simulink model "lqr_tracking_backup"  (R2017a)
settings: Solver=ode5  StartTime=0.0  StopTime=50  FixedStep=Ts  RelTol=1e-3  EnableMultiTasking=on
values from neighbouring files (symbols this model uses):
  Ki_lqr = [0 0 0.1 0 0 -0.1 0 0 8.66025403784 0 0 0 ... (16 elements, 4x4)]    [K_lqr.mat]
  Kx_lqr = [0 0 0.263619393691 0 0 -0.257300038922 0 0 13.6588017709 0 0 0 ... (48 elements, 4x12)]    [K_lqr.mat]
undefined symbols (not defined in the file or in its folder): B_ENU_inv, gra, KT, mass, sigbuilder_block
settings Model: Creator=dtnguyen  LastModifiedBy=ducnguyen
settings DataIOCC: LimitDataPoints=on  SaveFormat=Array
settings OptimizationCC: DefaultParameterBehavior=Inlined  UseFloatMulNetSlope=on  InlineInvariantSignals=on  PassReuseOutputArgsThreshold=0  EfficientFloat2IntCast=on
settings DebuggingCC: ParameterTunabilityLossMsg=error  SFUnexpectedBacktrackingDiag=warning  SFNoUnconditionalDefaultTransitionDiag=warning  SFExecutionAtInitializationDiag=none
settings HardwareCC: ProdBitPerPointer=32  ProdBitPerSizeT=32  ProdBitPerPtrDiffT=32  ProdLargestAtomicFloat=None  ProdIntDivRoundTo=Undefined  ProdEndianess=Unspecified  ProdWordSize=32  ProdHWDeviceType=32-bit Generic
settings ModelReferenceCC: PropagateSignalLabelsOutOfModel=off
settings RTWCC: PackageGeneratedCodeAndArtifacts=on  PackageName=myCodeExport  GenerateReport=on  Toolchain=Catkin  BuildConfiguration=Faster Runs  LaunchReport=on  TargetLang=C++  CheckMdlBeforeBuild=Warning
settings CodeAppCC: ForceParamTrailComments=on  OperatorAnnotations=on  MATLABSourceComments=on
settings GRTTargetCC: TargetLangStandard=C++03 (ISO)  MatFileLogging=off  MultiInstanceERTCode=on  CodeInterfacePackaging=C++ class
settings ConfigComp: CovMetricSettings=dw  CovHtmlReporting=on  CovSaveCumulativeToWorkspaceVar=on  CovSaveSingleToWorkspaceVar=on  CovExternalEMLEnable=off

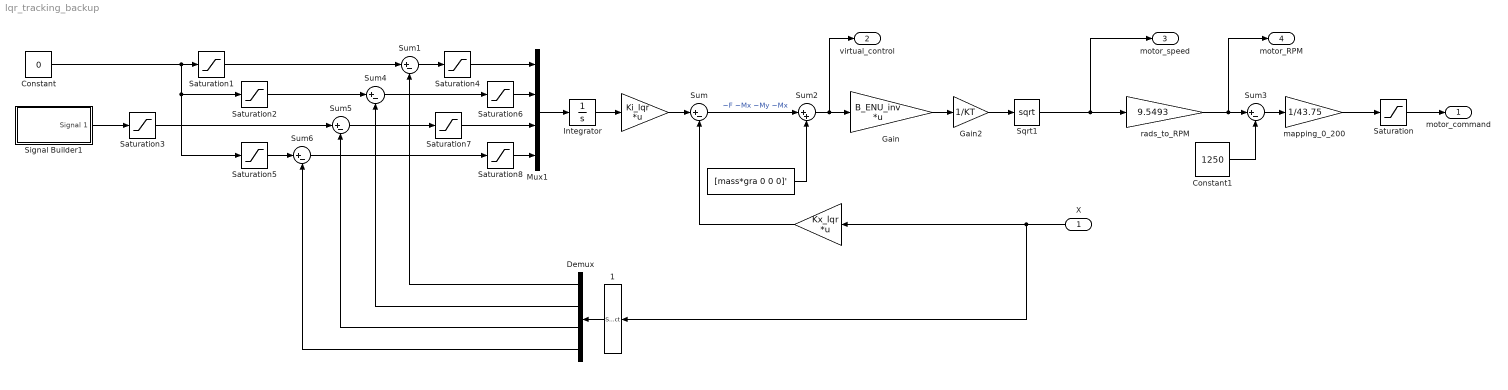
== system lqr_tracking_backup ==
  X : Inport  PortDimensions=12
  " " : Gain  Gain=Ki_lqr  Multiplication=Matrix(K*u)
  "              " : Constant  Value=[mass*gra 0 0 0]'
  "                   " : Gain  Gain=Kx_lqr  Multiplication=Matrix(K*u)
  "                    1" : Selector  InputPortWidth=12  IndexOptions=Index vector (dialog)  Indices=[1 2 3 9]  OutputSizes=1
  Constant : Constant  Value=0
  Constant1 : Constant  Value=1250  VectorParams1D=off  SampleTime=-1
  Demux : Demux
  Gain : Gain  Gain=B_ENU_inv  Multiplication=Matrix(K*u)
  Gain2 : Gain  Gain=1/KT
  Integrator : Integrator  InitialCondition=[0 0 0 0]'
  Mux1 : Mux
  Saturation : Saturate  UpperLimit=200  LowerLimit=0
  Saturation1 : Saturate  UpperLimit=2  LowerLimit=-2
  Saturation2 : Saturate  UpperLimit=2  LowerLimit=-2
  Saturation3 : Saturate  UpperLimit=1.75  LowerLimit=0
  Saturation4 : Saturate  UpperLimit=1  LowerLimit=-1
  Saturation5 : Saturate  UpperLimit=2*pi  LowerLimit=-2*pi
  Saturation6 : Saturate  UpperLimit=1  LowerLimit=-1
  Saturation7 : Saturate
  Saturation8 : Saturate  UpperLimit=pi/4  LowerLimit=-pi/4
  Signal Builder1 : Subsystem  Tag=STV Subsys  LoadFcn=sigbuilder_block('load');  StartFcn=sigbuilder_block('start');  StopFcn=sigbuilder_block('stop');  ClipboardFcn=sigbuilder_block('clipboard');  mask(Sigbuilder block){tuvar=[0:10]}
      mask help: Simulink:masks:SigbuilderBlock_MD
      mask init:
      | if ~strcmp(get_param(bdroot(gcbh),'SimulationStatus'),'stopped') tuvar = sigbuilder_block('maskInit'); end
      settings: CopyFcn=sigbuilder_block('copy');  DeleteFcn=sigbuilder_block('delete');  ModelCloseFcn=sigbuilder_block('modelClose');  PreSaveFcn=sigbuilder_block('preSave');  PauseFcn=sigbuilder_block('pause');  ContinueFcn=sigbuilder_block('continue');  NameChangeFcn=sigbuilder_block('namechange');  OpenFcn=sigbuilder_block('open',[425.25 198.75 556.5 403.5 ]);  CloseFcn=sigbuilder_block('close');
      mask Display: plot(0, 0, 100, 100,[2, 2, 32, 32, 2], [68, 8, 8, 68, 68],[32, 2], [38, 38], [32, 19, 2],[53, 60, 44], [32, 17, 17, 2],[16, 16, 31, 31]);txt = getActiveGroup(gcbh);text(2, 100, txt,'verticalAlignment', 'top');
  Sqrt1 : Sqrt  SaturateOnIntegerOverflow=on
  Sum{,1,3..6} (6 alike) : Sum  Inputs=|+-
  Sum2 : Sum  Inputs=|++
  mapping_0_200 : Gain  Gain=1/43.75
  rads_to_RPM : Gain  Gain=9.5493
  motor_command : Outport  PortDimensions=6
  virtual_control : Outport  Port=2  PortDimensions=4
  motor_speed : Outport  Port=3  PortDimensions=6
  motor_RPM : Outport  Port=4  PortDimensions=6
  wires:
  Gain2/1 -> Sqrt1/1
  X/1 -> "                   "/1, "                    1"/1
  Mux1/1 -> Integrator/1
  " "/1 -> Sum/1
  Integrator/1 -> " "/1
  "                   "/1 -> Sum/2
  Gain/1 -> Gain2/1
  Sum2/1 -> Gain/1, virtual_control/1
  Sum/1 -> Sum2/1  "~F ~Mx ~My ~Mx"
  "              "/1 -> Sum2/2
  Constant1/1 -> Sum3/2
  rads_to_RPM/1 -> Sum3/1, motor_RPM/1
  Sum3/1 -> mapping_0_200/1
  mapping_0_200/1 -> Saturation/1
  Saturation/1 -> motor_command/1
  Saturation1/1 -> Sum1/1
  Sum1/1 -> Saturation4/1
  Sum4/1 -> Saturation6/1
  Sum5/1 -> Saturation7/1
  Sum6/1 -> Saturation8/1
  "                    1"/1 -> Demux/1
  Demux/1 -> Sum1/2
  Demux/2 -> Sum4/2
  Demux/3 -> Sum5/2
  Demux/4 -> Sum6/2
  Saturation2/1 -> Sum4/1
  Saturation3/1 -> Sum5/1
  Constant/1 -> Saturation1/1, Saturation5/1, Saturation2/1
  Saturation4/1 -> Mux1/1
  Saturation5/1 -> Sum6/1
  Saturation6/1 -> Mux1/2
  Saturation7/1 -> Mux1/3
  Saturation8/1 -> Mux1/4
  Sqrt1/1 -> rads_to_RPM/1, motor_speed/1
  Signal Builder1/1(Signal 1) -> Saturation3/1

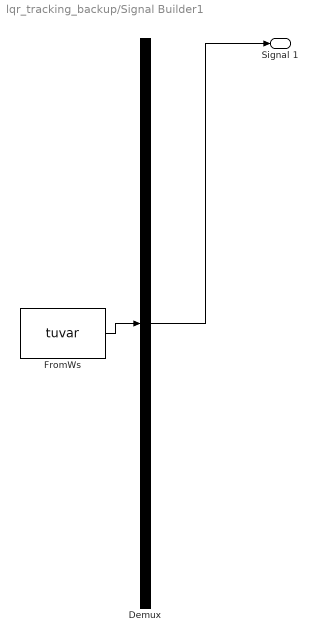
== system lqr_tracking_backup/Signal Builder1 ==
  Demux : Demux  Tag=STV Demux  Outputs=1
  FromWs : FromWorkspace  Tag=STV FromWs  VariableName=tuvar  SampleTime=0
      SigBuilderData=|
      | common.afterFinalStr = 'Extrapolate'
      | common.sampleTime = 0
      | dataSet.timeRange = [0 20]
      | dataSet.name = 'Group 1'
      | sbobj.Groups.Name = 'Group 1'
      | sbobj.Groups.Signals.Name = 'Signal 1'
      | sbobj.Groups.Signals.XData = [0 2.5 17.5 20]
      | sbobj.Groups.Signals.YData = [0 0.5 0.5 0]
      | sbobj.Groups.TimeRange = [0 20]
  Signal 1 : Outport  Tag=STV Outport
  wires:
  Demux/1 -> Signal 1/1
  FromWs/1 -> Demux/1
